simulink model "lixo"  (R2017b)
settings: Solver=VariableStepAuto  StartTime=0.0  StopTime=20  MaxStep=1e-3  RelTol=1e-6  AbsTol=1e-3
undefined symbols (not defined in the file): ssPitch
settings Model: Creator=PauloOliveira  LastModifiedBy=PauloOliveira

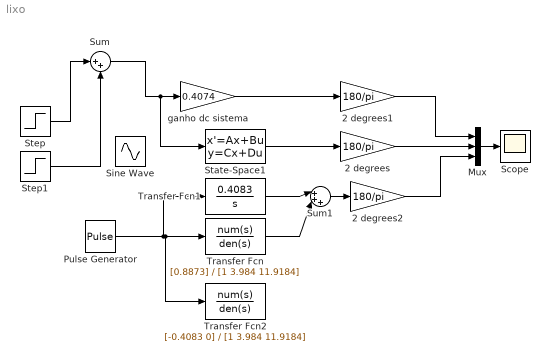
== system lixo ==
  2 degrees : Gain  Gain=180/pi
  2 degrees1 : Gain  Gain=180/pi
  2 degrees2 : Gain  Gain=180/pi
  Mux : Mux  Inputs=3
  Pulse Generator : DiscretePulseGenerator  PulseType=Time based  Amplitude=100  Period=100  PulseWidth=2*10/10000  PhaseDelay=10
  Scope : Scope
  Sine Wave : Sin  Frequency=1.9357  SampleTime=0
  State-Space1 : StateSpace  A=ssPitch.a  B=ssPitch.b  C=ssPitch.c  D=ssPitch.d  InitialCondition=0
  Step : Step  Time=10  After=0.2  SampleTime=0
  Step1 : Step  Time=13.5  After=-0.2  SampleTime=0
  Sum : Sum  Inputs=|++
  Sum1 : Sum  Inputs=|+++
  Transfer Fcn : TransferFcn  Numerator=[0.8873]  Denominator=[1 3.984 11.9184]
  Transfer Fcn1 : TransferFcn  Numerator=[0.4083]  Denominator=[1 0]
  Transfer Fcn2 : TransferFcn  Numerator=[-0.4083 0]  Denominator=[1 3.984 11.9184]
  "ganho dc sistema " : Gain  Gain=0.4074
  wires:
  State-Space1/1 -> 2 degrees/1
  Step/1 -> Sum/1
  Step1/1 -> Sum/2
  Mux/1 -> Scope/1
  2 degrees/1 -> Mux/2
  2 degrees1/1 -> Mux/1
  "ganho dc sistema "/1 -> 2 degrees1/1
  Transfer Fcn1/1 -> Sum1/1
  Transfer Fcn/1 -> Sum1/2
  Sum1/1 -> 2 degrees2/1
  2 degrees2/1 -> Mux/3
  Pulse Generator/1 -> Transfer Fcn2/1, Transfer Fcn/1, Transfer Fcn1/1
  Sum/1 -> State-Space1/1, "ganho dc sistema "/1
